simulink library "csc_pcs_power_control_system_lib"  (R2014b)
settings: Solver=ode113  StartTime=0.0  StopTime=10.0  RelTol=1e-3
values from neighbouring files (symbols this model uses):
  fsw_dt = 0.1    [csu_cmv_convert_measured_voltages_collection_test.m]
libraries: util_common_lib x2, util_info_lib x1, csu_cmc_convert_measured_currents_collection_lib x1, csu_cmv_convert_measured_voltages_collection_lib x1
settings Model: Creator=Jim Kaidy  LastModifiedBy=mstewart

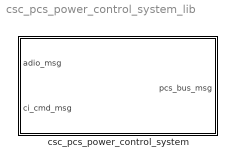
== system csc_pcs_power_control_system_lib ==
  csc_pcs_power_control_system : Subsystem  Tag=OFSW; MDL_TICK=ADIO_MSG  TreatAsAtomicUnit=on  SystemSampleTime=fsw_dt

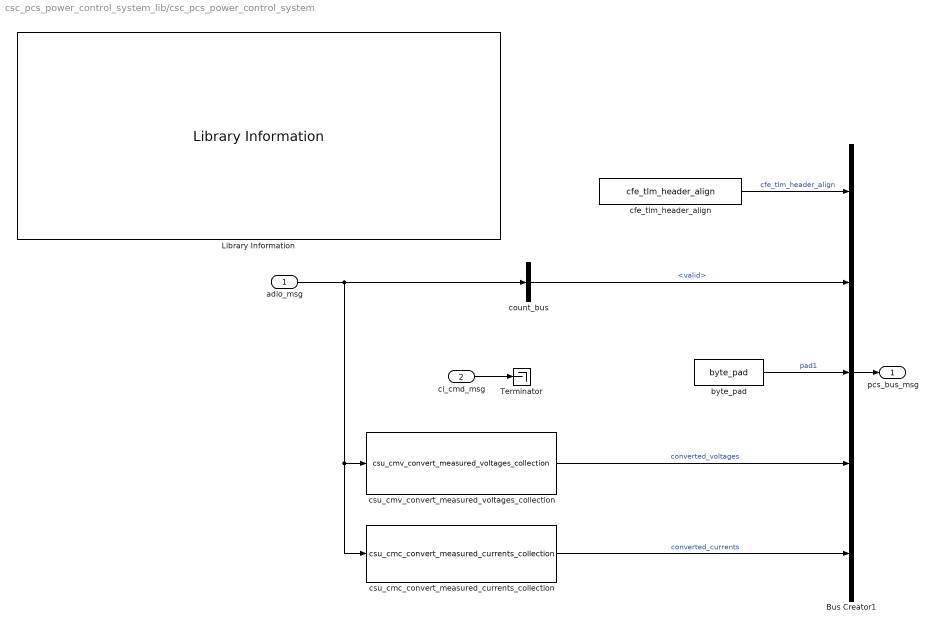
== system csc_pcs_power_control_system_lib/csc_pcs_power_control_system ==
  adio_msg : Inport
  ci_cmd_msg : Inport  Port=2
  Bus Creator1 : BusCreator  Inputs=5  OutDataTypeStr=Bus: pcs_bus_msg  NonVirtualBus=on
  Library Information : util_info_lib/Library Information  owner='escrane'
  Terminator : Terminator
  byte_pad : util_common_lib/byte_pad  n_bytes=7
  cfe_tlm_header_align : util_common_lib/cfe_tlm_header_align
  count_bus : BusSelector  OutputSignals=valid
  csu_cmc_convert_measured_currents_collection : csu_cmc_convert_measured_currents_collection_lib/csu_cmc_convert_measured_currents_collection  SystemSampleTime=-1
  csu_cmv_convert_measured_voltages_collection : csu_cmv_convert_measured_voltages_collection_lib/csu_cmv_convert_measured_voltages_collection  SystemSampleTime=-1
  pcs_bus_msg : Outport  OutDataTypeStr=Bus: pcs_bus_msg
  wires:
  count_bus/1 -> Bus Creator1/2  "<valid>"
  byte_pad/1 -> Bus Creator1/3  "pad1"
  cfe_tlm_header_align/1 -> Bus Creator1/1  "cfe_tlm_header_align"
  ci_cmd_msg/1 -> Terminator/1
  Bus Creator1/1 -> pcs_bus_msg/1
  adio_msg/1 -> count_bus/1, csu_cmc_convert_measured_currents_collection/1, csu_cmv_convert_measured_voltages_collection/1
  csu_cmv_convert_measured_voltages_collection/1 -> Bus Creator1/4  "converted_voltages"
  csu_cmc_convert_measured_currents_collection/1 -> Bus Creator1/5  "converted_currents"
